simulink model "rct_airframe2"  (R2023a)
settings: Solver=ode23t  StartTime=0.0  StopTime=5  RelTol=1e-3  AbsTol=1e-6
model workspace (MAT data in the model file):
  Beamwidth = 0.174532925199
  Cm_alpha = [7.78  6.42  5.06  3.7  2.34; 7.179815  5.887815  4.595815  3.303815  2.011815; 6.59412  5.37012  4.14612  2.92212  1.69812; 6.024205  4.868205  3.712205  2.556205  1.400205; 5.47136  4.38336  3.29536  2.20736  1.11936; 4.936875  3.916875  2.896875  1.876875  0.856875; 4.42204  3.47004  2.51804  1.56604  0.61404; 3.928145  3.044145  2.160145  1.276145  0.392145; 3.45648  2.64048  1.82448  1.00848  0.19248; 3.008335  2.260335  1.512335  0.764335  0.016335; 2.585  1.905  1.225  0.545  -0.135; 2.187765  1.575765  0.963765  0.351765  -0.260235; 1.81792  1.27392  0.72992  0.18592  -0.35808; 1.476755  1.000755  0.524755  0.048755  -0.427245; 1.16556  0.75756  0.34956  -0.05844  -0.46644; 0.885625  0.545625  0.205625  -0.134375  -0.474375; 0.63824  0.36624  0.09424  -0.17776  -0.44976; 0.424695  0.220695  0.016695  -0.187305  -0.391305; 0.24628  0.11028  -0.02572  -0.16172  -0.29772; 0.104285  0.036285  -0.031715  -0.099715  -0.167715; 0  0  0  0  0; -0.104285  -0.036285  0.031715  0.099715  0.167715; -0.24628  -0.11028  0.02572  0.16172  0.29772; -0.424695  -0.220695  -0.016695  0.187305  0.391305; -0.63824  -0.36624  -0.09424  0.17776  0.44976; -0.885625  -0.545625  -0.205625  0.134375  0.474375; -1.16556  -0.75756  -0.34956  0.05844  0.46644; -1.476755  -1.000755  -0.524755  -0.048755  0.427245; -1.81792  -1.27392  -0.72992  -0.18592  0.35808; -2.187765  -1.575765  -0.963765  -0.351765  0.260235; -2.585  -1.905  -1.225  -0.545  0.135; -3.008335  -2.260335  -1.512335  -0.764335  -0.016335; -3.45648  -2.64048  -1.82448  -1.00848  -0.19248; -3.928145  -3.044145  -2.160145  -1.276145  -0.392145; -4.42204  -3.47004  -2.51804  -1.56604  -0.61404; -4.936875  -3.916875  -2.896875  -1.876875  -0.856875; -5.47136  -4.38336  -3.29536  -2.20736  -1.11936; -6.024205  -4.868205  -3.712205  -2.556205  -1.400205; -6.59412  -5.37012  -4.14612  -2.92212  -1.69812; -7.179815  -5.887815  -4.595815  -3.303815  -2.011815; -7.78  -6.42  -5.06  -3.7  -2.34]
  Cm_el = -11.8029305797
  Cm_q = -1.719
  Cx_alpha = [-0.3  -0.3  -0.3  -0.3  -0.3; -0.3  -0.3  -0.3  -0.3  -0.3; -0.3  -0.3  -0.3  -0.3  -0.3; -0.3  -0.3  -0.3  -0.3  -0.3; -0.3  -0.3  -0.3  -0.3  -0.3; -0.3  -0.3  -0.3  -0.3  -0.3; -0.3  -0.3  -0.3  -0.3  -0.3; -0.3  -0.3  -0.3  -0.3  -0.3; -0.3  -0.3  -0.3  -0.3  -0.3; -0.3  -0.3  -0.3  -0.3  -0.3; -0.3  -0.3  -0.3  -0.3  -0.3; -0.3  -0.3  -0.3  -0.3  -0.3; -0.3  -0.3  -0.3  -0.3  -0.3; -0.3  -0.3  -0.3  -0.3  -0.3; -0.3  -0.3  -0.3  -0.3  -0.3; -0.3  -0.3  -0.3  -0.3  -0.3; -0.3  -0.3  -0.3  -0.3  -0.3; -0.3  -0.3  -0.3  -0.3  -0.3; -0.3  -0.3  -0.3  -0.3  -0.3; -0.3  -0.3  -0.3  -0.3  -0.3; -0.3  -0.3  -0.3  -0.3  -0.3; -0.3  -0.3  -0.3  -0.3  -0.3; -0.3  -0.3  -0.3  -0.3  -0.3; -0.3  -0.3  -0.3  -0.3  -0.3; -0.3  -0.3  -0.3  -0.3  -0.3; -0.3  -0.3  -0.3  -0.3  -0.3; -0.3  -0.3  -0.3  -0.3  -0.3; -0.3  -0.3  -0.3  -0.3  -0.3; -0.3  -0.3  -0.3  -0.3  -0.3; -0.3  -0.3  -0.3  -0.3  -0.3; -0.3  -0.3  -0.3  -0.3  -0.3; -0.3  -0.3  -0.3  -0.3  -0.3; -0.3  -0.3  -0.3  -0.3  -0.3; -0.3  -0.3  -0.3  -0.3  -0.3; -0.3  -0.3  -0.3  -0.3  -0.3; -0.3  -0.3  -0.3  -0.3  -0.3; -0.3  -0.3  -0.3  -0.3  -0.3; -0.3  -0.3  -0.3  -0.3  -0.3; -0.3  -0.3  -0.3  -0.3  -0.3; -0.3  -0.3  -0.3  -0.3  -0.3; -0.3  -0.3  -0.3  -0.3  -0.3]
  Cz_alpha = [7.47866666667 7.00150633333 6.531504 6.06927766667 5.61544533333 5.170625 4.73543466667 4.31049233333 3.896416 3.49382366667 3.10333333333 2.725563 ... (205 elements, 41x5)]
  Cz_el = -1.94805650344
  Iyy = 247.436636441
  K_r = -0.02
  Kg2slug = 0.0685218
  Ks = 125.663706144
  L = 0.0065
  M = [2  2.5  3  3.5  4; 2  2.5  3  3.5  4; 2  2.5  3  3.5  4; 2  2.5  3  3.5  4; 2  2.5  3  3.5  4; 2  2.5  3  3.5  4; 2  2.5  3  3.5  4; 2  2.5  3  3.5  4; 2  2.5  3  3.5  4; 2  2.5  3  3.5  4; 2  2.5  3  3.5  4; 2  2.5  3  3.5  4; 2  2.5  3  3.5  4; 2  2.5  3  3.5  4; 2  2.5  3  3.5  4; 2  2.5  3  3.5  4; 2  2.5  3  3.5  4; 2  2.5  3  3.5  4; 2  2.5  3  3.5  4; 2  2.5  3  3.5  4; 2  2.5  3  3.5  4; 2  2.5  3  3.5  4; 2  2.5  3  3.5  4; 2  2.5  3  3.5  4; 2  2.5  3  3.5  4; 2  2.5  3  3.5  4; 2  2.5  3  3.5  4; 2  2.5  3  3.5  4; 2  2.5  3  3.5  4; 2  2.5  3  3.5  4; 2  2.5  3  3.5  4; 2  2.5  3  3.5  4; 2  2.5  3  3.5  4; 2  2.5  3  3.5  4; 2  2.5  3  3.5  4; 2  2.5  3  3.5  4; 2  2.5  3  3.5  4; 2  2.5  3  3.5  4; 2  2.5  3  3.5  4; 2  2.5  3  3.5  4; 2  2.5  3  3.5  4]
  Mach_vec = [2 2.5 3 3.5 4]
  P0 = 101325
  R = 287.26
  S_ref = 0.0408773349839
  T0 = 288.16
  Thrust = 10000
  al = [-20  -20  -20  -20  -20; -19  -19  -19  -19  -19; -18  -18  -18  -18  -18; -17  -17  -17  -17  -17; -16  -16  -16  -16  -16; -15  -15  -15  -15  -15; -14  -14  -14  -14  -14; -13  -13  -13  -13  -13; -12  -12  -12  -12  -12; -11  -11  -11  -11  -11; -10  -10  -10  -10  -10; -9  -9  -9  -9  -9; -8  -8  -8  -8  -8; -7  -7  -7  -7  -7; -6  -6  -6  -6  -6; -5  -5  -5  -5  -5; -4  -4  -4  -4  -4; -3  -3  -3  -3  -3; -2  -2  -2  -2  -2; -1  -1  -1  -1  -1; 0  0  0  0  0; 1  1  1  1  1; 2  2  2  2  2; 3  3  3  3  3; 4  4  4  4  4; 5  5  5  5  5; 6  6  6  6  6; 7  7  7  7  7; 8  8  8  8  8; 9  9  9  9  9; 10  10  10  10  10; 11  11  11  11  11; 12  12  12  12  12; 13  13  13  13  13; 14  14  14  14  14; 15  15  15  15  15; 16  16  16  16  16; 17  17  17  17  17; 18  18  18  18  18; 19  19  19  19  19; 20  20  20  20  20]
  alpha_ini = 0
  alpha_vec = [-0.349065850399; -0.331612557879; -0.314159265359; -0.296705972839; -0.279252680319; -0.261799387799; -0.244346095279; -0.226892802759; -0.209439510239; -0.191986217719; -0.174532925199; -0.157079632679; -0.13962634016; -0.12217304764; -0.10471975512; -0.0872664625997; -0.0698131700798; -0.0523598775598; -0.0349065850399; -0.0174532925199; 0; 0.0174532925199; 0.0349065850399; 0.0523598775598; 0.0698131700798; 0.0872664625997; 0.10471975512; 0.12217304764; 0.13962634016; 0.157079632679; 0.174532925199; 0.191986217719; 0.209439510239; 0.226892802759; 0.244346095279; 0.261799387799; 0.279252680319; 0.296705972839; 0.314159265359; 0.331612557879; 0.349065850399]
  am = 0.000215
  an = 0.000103
  bm = -0.0195
  bn = -0.00945
  cm = 0.051
  cn = -0.1696
  d2r = 0.0174532925199
  d_ref = 0.228599992685
  fin_act_0 = 0
  fin_max = 0.523598775598
  fin_maxrate = 8.72664625997
  fin_min = -0.523598775598
  g = 9.81
  gam = 1.403
  h_ini = 3047.99990246
  h_trop = 11000
  l_acc = 0.5
  m2ft = 3.28084
  mass = 204.022661401
  max_gimbal = 0.610865238198
  min_gimbal = -0.610865238198
  pos_tgt = [4500 -3547.99990246]
  q_ini = 0
  rho0 = 1.225
  theta_ini = 0
  theta_tgt = 3.14159265359
  tors = 0.05
  v_ini = 984
  v_tgt = 328
  wgyro = 628.318530718
  wn_fin = 150
  wn_hom = 7
  x_ini = 0
  z_fin = 0.7
libraries: aerospace x3
settings Model: ExtModeTrigMode=oneshot  Creator=The MathWorks, Inc.  LastModifiedBy=The MathWorks, Inc.
settings SolverCC: AutoScaleAbsTol=off  AlgebraicLoopSolver=TrustRegion
settings DataIOCC: SaveFormat=Array  SaveOutput=off  SignalLogging=off  SaveTime=off  ReturnWorkspaceOutputs=off  SignalLoggingName=sigsOut
settings OptimizationCC: BlockReduction=off  BooleanDataType=off  DefaultParameterBehavior=Inlined  InlineInvariantSignals=on  BufferReuse=off  ExpressionDepthLimit=2147483647  InitFltsAndDblsToZero=on  LifeSpan=inf
settings DebuggingCC: SaveWithParameterizedLinksMsg=none  UnderspecifiedInitializationDetection=Classic  MergeDetectMultiDrivingBlocksExec=none  CheckExecutionContextPreStartOutputMsg=on  SignalResolutionControl=TryResolveAllWithWarning  MultiTaskDSMMsg=warning  FcnCallInpInsideContextMsg=warning  UnconnectedInputMsg=warning  UnconnectedOutputMsg=warning  UnconnectedLineMsg=warning  AllowSymbolicDim=off  StateNameClashWarn=warning  SFUnexpectedBacktrackingDiag=warning  SFNoUnconditionalDefaultTransitionDiag=warning  ArithmeticOperatorsInVariantConditions=warning
settings HardwareCC: ProdBitPerPointer=32  ProdBitPerSizeT=32  ProdBitPerPtrDiffT=32  ProdLargestAtomicFloat=None  ProdIntDivRoundTo=Undefined  ProdEndianess=Unspecified  ProdWordSize=32  ProdHWDeviceType=32-bit Generic  TargetUnknown=on
settings ModelReferenceCC: UpdateModelReferenceTargets=IfOutOfDate  EnableRefExpFcnMdlSchedulingChecks=on  PropagateSignalLabelsOutOfModel=off
settings SFSimCC: SimUseLocalCustomCode=off  CustomCodeUndefinedFunction=UseInterfaceOnly
settings RTWCC: RTWUseLocalCustomCode=off  DLArmComputeVersion=19.05
settings CodeAppCC: StateflowObjectComments=on
settings GRTTargetCC: TargetFcnLib=ansi_tfl_tmw.mat  TargetLangStandard=C89/C90 (ANSI)  CombineOutputUpdateFcns=off  GRTInterface=on
settings ConfigComp: CovMetricSettings=dw  CovSaveCumulativeToWorkspaceVar=on  CovSaveSingleToWorkspaceVar=on  CovExternalEMLEnable=off  CovSFcnEnable=off

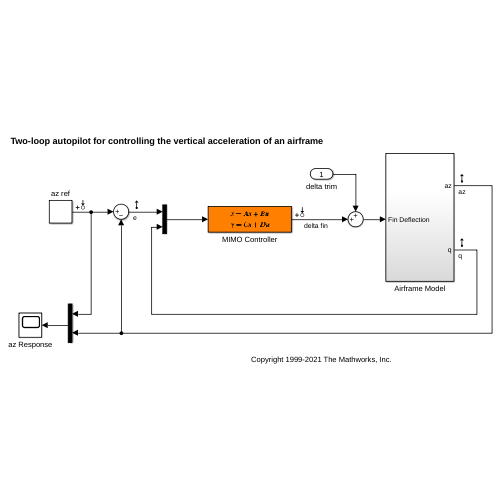
[thumbnail: Simulink's stored preview of the top-level diagram]
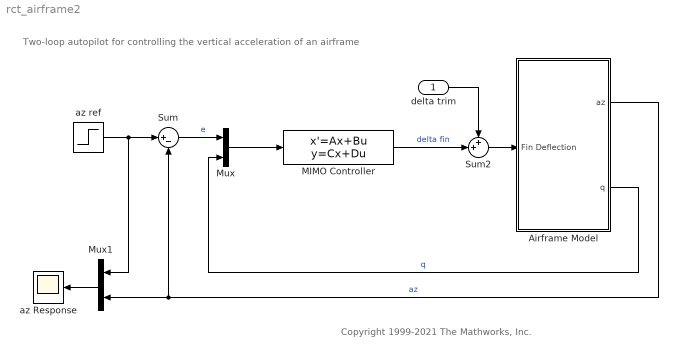
== system rct_airframe2 ==
  note: Copyright 1999-2021 The Mathworks, Inc.
  note: Two-loop autopilot for controlling the vertical acceleration of an airframe
  delta trim : Inport
  Airframe Model : Subsystem
      settings: RTWMemSecFuncInitTerm=Default  RTWMemSecFuncExecute=Default  RTWMemSecDataConstants=Default  RTWMemSecDataInternal=Default  RTWMemSecDataParameters=Default
  MIMO Controller : StateSpace  A=[0 0.08;0 0]  B=[0.003 1;0.125 0]  C=[1.5 0]  D=[0 0]  InitialCondition=0
  Mux : Mux  Inputs=2
  Mux1 : Mux  Inputs=2
  Sum : Sum  Inputs=|+-  SaturateOnIntegerOverflow=on
  Sum2 : Sum  Inputs=++|
  az Response : Scope
  az ref : Step  After=200  SampleTime=0
  wires:
  Sum/1 -> Mux/1  "e"
  Mux1/1 -> az Response/1
  az ref/1 -> Sum/1, Mux1/1
  Airframe Model/1(az) -> Mux1/2, Sum/2  "az"
  Airframe Model/2(q) -> Mux/2  "q"
  Mux/1 -> MIMO Controller/1
  MIMO Controller/1 -> Sum2/2  "delta fin"
  Sum2/1 -> Airframe Model/1(Fin Deflection)
  delta trim/1 -> Sum2/1

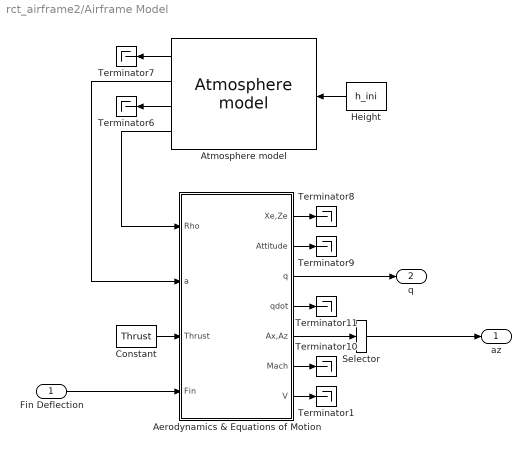
== system rct_airframe2/Airframe Model ==
  Fin Deflection : Inport
  Aerodynamics & Equations of Motion : Subsystem
      settings: RTWMemSecFuncInitTerm=Default  RTWMemSecFuncExecute=Default  RTWMemSecDataConstants=Default  RTWMemSecDataInternal=Default  RTWMemSecDataParameters=Default
  Atmosphere model : aerospace/Atmosphere/Atmosphere model
  Constant : Constant  Value=Thrust
  Height : Constant  Value=h_ini
  Selector : Selector  InputPortWidth=2  IndexOptions=Index vector (dialog)  Indices=[2]  OutputSizes=1
  Terminator{1,6..11} (7 alike) : Terminator
  az : Outport  InitialOutput=0
  q : Outport  Port=2  InitialOutput=0
  wires:
  Height/1 -> Atmosphere model/1
  Atmosphere model/1 -> Terminator7/1
  Atmosphere model/3 -> Terminator6/1
  Constant/1 -> Aerodynamics & Equations of Motion/3(Thrust)
  Fin Deflection/1 -> Aerodynamics & Equations of Motion/4(Fin)
  Aerodynamics & Equations of Motion/1(Xe,Ze) -> Terminator8/1
  Aerodynamics & Equations of Motion/2(Attitude) -> Terminator9/1
  Aerodynamics & Equations of Motion/3(q) -> q/1
  Aerodynamics & Equations of Motion/4(qdot) -> Terminator11/1
  Aerodynamics & Equations of Motion/5(Ax,Az) -> Selector/1
  Aerodynamics & Equations of Motion/6(Mach) -> Terminator10/1
  Atmosphere model/4 -> Aerodynamics & Equations of Motion/1(Rho)
  Atmosphere model/2 -> Aerodynamics & Equations of Motion/2(a)
  Selector/1 -> az/1
  Aerodynamics & Equations of Motion/7(V) -> Terminator1/1

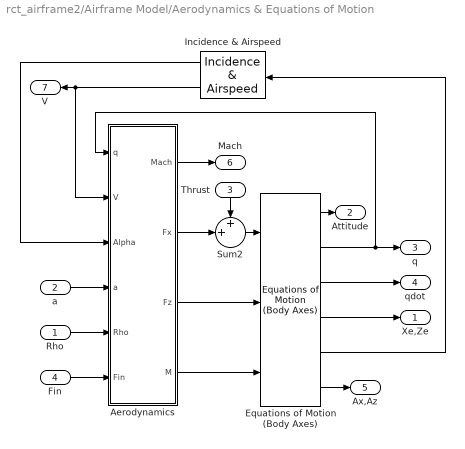
== system rct_airframe2/Airframe Model/Aerodynamics & Equations of Motion ==
  Rho : Inport
  a : Inport  Port=2
  Thrust : Inport  Port=3
  Fin : Inport  Port=4
  " Equations of Motion (Body Axes)" : aerospace/3DoF Equations of Motion / Equations of Motion (Body Axes)  v_ini=v_ini  theta_ini=theta_ini  alpha_ini=alpha_ini  q_ini=q_ini  pos_ini=[x_ini -h_ini]  mass=mass  Iyy=Iyy  g=g
  Aerodynamics : Subsystem
      settings: RTWMemSecFuncInitTerm=Default  RTWMemSecFuncExecute=Default  RTWMemSecDataConstants=Default  RTWMemSecDataInternal=Default  RTWMemSecDataParameters=Default
  Incidence & Airspeed : aerospace/3DoF Equations of Motion /Incidence  & Airspeed
  Sum2 : Sum  Inputs=++|  InputSameDT=on  SaturateOnIntegerOverflow=on  OutDataTypeStr=Inherit: Same as first input
  Xe,Ze : Outport  InitialOutput=0
  Attitude : Outport  Port=2  InitialOutput=0
  q : Outport  Port=3  InitialOutput=0
  qdot : Outport  Port=4  InitialOutput=0
  Ax,Az : Outport  Port=5  InitialOutput=0
  Mach : Outport  Port=6  InitialOutput=0
  V : Outport  Port=7  InitialOutput=0
  wires:
  " Equations of Motion (Body Axes)"/5 -> Incidence & Airspeed/1
  " Equations of Motion (Body Axes)"/6 -> Ax,Az/1
  " Equations of Motion (Body Axes)"/4 -> Xe,Ze/1
  " Equations of Motion (Body Axes)"/1 -> Attitude/1
  " Equations of Motion (Body Axes)"/3 -> qdot/1
  " Equations of Motion (Body Axes)"/2 -> Aerodynamics/1(q), q/1
  Thrust/1 -> Sum2/1
  Aerodynamics/2(Fx) -> Sum2/2
  Aerodynamics/3(Fz) -> " Equations of Motion (Body Axes)"/2
  Incidence & Airspeed/2 -> Aerodynamics/2(V), V/1
  Fin/1 -> Aerodynamics/6(Fin)
  a/1 -> Aerodynamics/4(a)
  Rho/1 -> Aerodynamics/5(Rho)
  Incidence & Airspeed/1 -> Aerodynamics/3(Alpha)
  Sum2/1 -> " Equations of Motion (Body Axes)"/1
  Aerodynamics/4(" M") -> " Equations of Motion (Body Axes)"/3
  Aerodynamics/1(" Mach") -> Mach/1

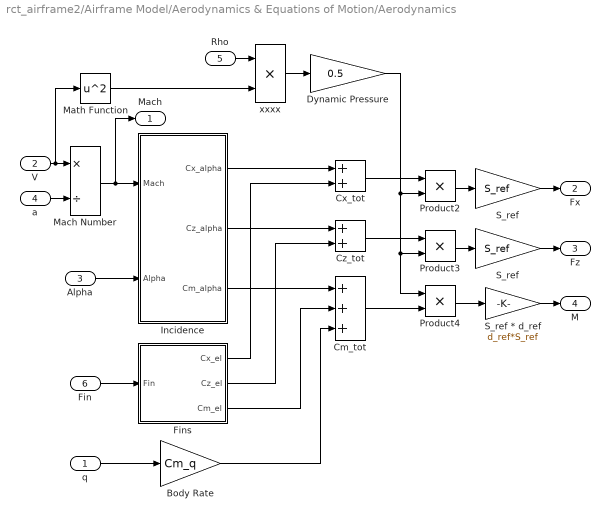
== system rct_airframe2/Airframe Model/Aerodynamics & Equations of Motion/Aerodynamics ==
  q : Inport
  V : Inport  Port=2
  Alpha : Inport  Port=3
  a : Inport  Port=4
  Rho : Inport  Port=5
  Fin : Inport  Port=6
  Body Rate : Gain  Gain=Cm_q  SaturateOnIntegerOverflow=on  OutDataTypeStr=Inherit: Same as input  ParamDataTypeStr=Inherit: Same as input
  Cm_tot : Sum  Inputs=+++  InputSameDT=on  SaturateOnIntegerOverflow=on  OutDataTypeStr=Inherit: Same as first input
  Cx_tot : Sum  InputSameDT=on  SaturateOnIntegerOverflow=on  OutDataTypeStr=Inherit: Same as first input
  Cz_tot : Sum  InputSameDT=on  SaturateOnIntegerOverflow=on  OutDataTypeStr=Inherit: Same as first input
  Dynamic Pressure : Gain  Gain=0.5  SaturateOnIntegerOverflow=on  OutDataTypeStr=Inherit: Same as input  ParamDataTypeStr=Inherit: Same as input
  Fins : Subsystem
      settings: RTWMemSecFuncInitTerm=Default  RTWMemSecFuncExecute=Default  RTWMemSecDataConstants=Default  RTWMemSecDataInternal=Default  RTWMemSecDataParameters=Default
  Incidence : Subsystem
      settings: RTWMemSecFuncInitTerm=Default  RTWMemSecFuncExecute=Default  RTWMemSecDataConstants=Default  RTWMemSecDataInternal=Default  RTWMemSecDataParameters=Default
  Mach Number : Product  Inputs=*/  InputSameDT=on  SaturateOnIntegerOverflow=on  OutDataTypeStr=Inherit: Same as first input
  Math Function : Math  Operator=square  SignedPower=on
  Product2 : Product  InputSameDT=on  SaturateOnIntegerOverflow=on  OutDataTypeStr=Inherit: Same as first input
  Product3 : Product  InputSameDT=on  SaturateOnIntegerOverflow=on  OutDataTypeStr=Inherit: Same as first input
  Product4 : Product  InputSameDT=on  SaturateOnIntegerOverflow=on  OutDataTypeStr=Inherit: Same as first input
  S_ref : Gain  Gain=S_ref  SaturateOnIntegerOverflow=on  OutDataTypeStr=Inherit: Same as input  ParamDataTypeStr=Inherit: Same as input
  S_ref * d_ref : Gain  Gain=d_ref*S_ref  SaturateOnIntegerOverflow=on  OutDataTypeStr=Inherit: Same as input  ParamDataTypeStr=Inherit: Same as input
  "S_ref " : Gain  Gain=S_ref  SaturateOnIntegerOverflow=on  OutDataTypeStr=Inherit: Same as input  ParamDataTypeStr=Inherit: Same as input
  xxxx : Product  InputSameDT=on  SaturateOnIntegerOverflow=on  OutDataTypeStr=Inherit: Same as first input
  " Mach" : Outport  InitialOutput=0
  Fx : Outport  Port=2  InitialOutput=[0]
  Fz : Outport  Port=3  InitialOutput=0
  " M" : Outport  Port=4  InitialOutput=0
  wires:
  Mach Number/1 -> Incidence/1(Mach), " Mach"/1
  q/1 -> Body Rate/1
  Cm_tot/1 -> Product4/2
  Product4/1 -> S_ref * d_ref/1
  S_ref * d_ref/1 -> " M"/1
  Fin/1 -> Fins/1(Fin)
  "S_ref "/1 -> Fz/1
  Product3/1 -> "S_ref "/1
  S_ref/1 -> Fx/1
  Product2/1 -> S_ref/1
  Cz_tot/1 -> Product3/1
  Cx_tot/1 -> Product2/1
  Alpha/1 -> Incidence/2(Alpha)
  a/1 -> Mach Number/2
  Body Rate/1 -> Cm_tot/3
  Fins/3(Cm_el) -> Cm_tot/2
  Incidence/3(Cm_alpha) -> Cm_tot/1
  Fins/2(Cz_el) -> Cz_tot/2
  Incidence/2(Cz_alpha) -> Cz_tot/1
  Fins/1(Cx_el) -> Cx_tot/2
  Incidence/1(Cx_alpha) -> Cx_tot/1
  V/1 -> Mach Number/1, Math Function/1
  Dynamic Pressure/1 -> Product4/1, Product3/2, Product2/2
  xxxx/1 -> Dynamic Pressure/1
  Rho/1 -> xxxx/1
  Math Function/1 -> xxxx/2

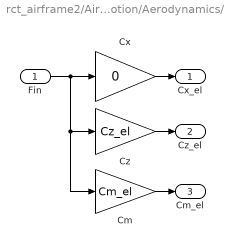
== system rct_airframe2/Airframe Model/Aerodynamics & Equations of Motion/Aerodynamics/Fins ==
  Fin : Inport
  Cm : Gain  Gain=Cm_el  SaturateOnIntegerOverflow=on  OutDataTypeStr=Inherit: Same as input  ParamDataTypeStr=Inherit: Same as input
  Cx : Gain  Gain=0  SaturateOnIntegerOverflow=on  OutDataTypeStr=Inherit: Same as input  ParamDataTypeStr=Inherit: Same as input
  Cz : Gain  Gain=Cz_el  SaturateOnIntegerOverflow=on  OutDataTypeStr=Inherit: Same as input  ParamDataTypeStr=Inherit: Same as input
  Cx_el : Outport  InitialOutput=0
  Cz_el : Outport  Port=2  InitialOutput=0
  Cm_el : Outport  Port=3  InitialOutput=0
  wires:
  Cz/1 -> Cz_el/1
  Cm/1 -> Cm_el/1
  Cx/1 -> Cx_el/1
  Fin/1 -> Cz/1, Cm/1, Cx/1

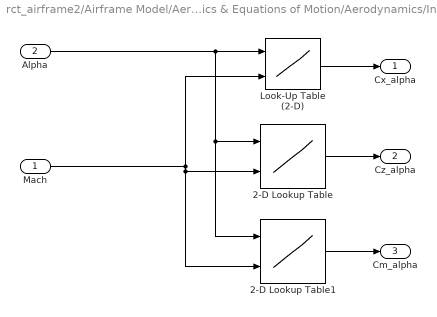
== system rct_airframe2/Airframe Model/Aerodynamics & Equations of Motion/Aerodynamics/Incidence ==
  Mach : Inport
  Alpha : Inport  Port=2
  2-D Lookup Table : Lookup_n-D  BreakpointsForDimension1=alpha_vec  BreakpointsForDimension2=Mach_vec  Table=Cz_alpha  RndMeth=Simplest
      settings: InputPortMap=u0,u1
  2-D Lookup Table1 : Lookup_n-D  BreakpointsForDimension1=alpha_vec  BreakpointsForDimension2=Mach_vec  Table=Cm_alpha  RndMeth=Simplest
      settings: InputPortMap=u0,u1
  Look-Up Table (2-D) : Lookup2D  RowIndex=alpha_vec  ColumnIndex=Mach_vec  Table=Cx_alpha  InputSameDT=off
  Cx_alpha : Outport  InitialOutput=0
  Cz_alpha : Outport  Port=2  InitialOutput=0
  Cm_alpha : Outport  Port=3  InitialOutput=0
  wires:
  Mach/1 -> 2-D Lookup Table1/2, 2-D Lookup Table/2, Look-Up Table (2-D)/2
  Alpha/1 -> 2-D Lookup Table1/1, 2-D Lookup Table/1, Look-Up Table (2-D)/1
  2-D Lookup Table1/1 -> Cm_alpha/1
  2-D Lookup Table/1 -> Cz_alpha/1
  Look-Up Table (2-D)/1 -> Cx_alpha/1
